simulink model "step_response_torque"  (R2024b)
settings: Solver=FixedStepAuto  StartTime=0.0  StopTime=10  FixedStep=Ts  RelTol=1e-3
values from neighbouring files (symbols this model uses):
  K_I = Ki_values(j)    [tune_PI_speed.m]
  K_p = Kp_values(i)    [tune_PI_speed.m]
  v0 = 10    [getItRunning.m]
libraries: slpidlib x1
settings Model: Creator=marti  LastModifiedBy=marti

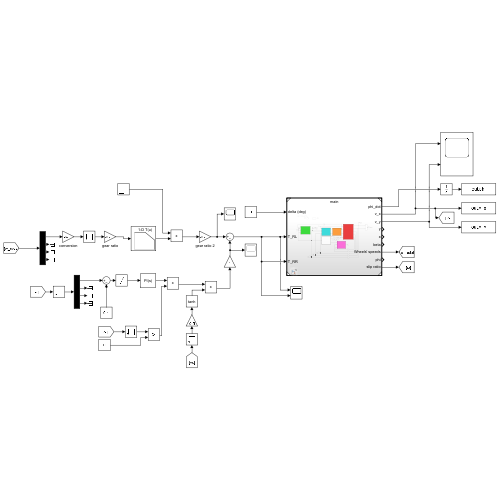
[thumbnail: Simulink's stored preview of the top-level diagram]
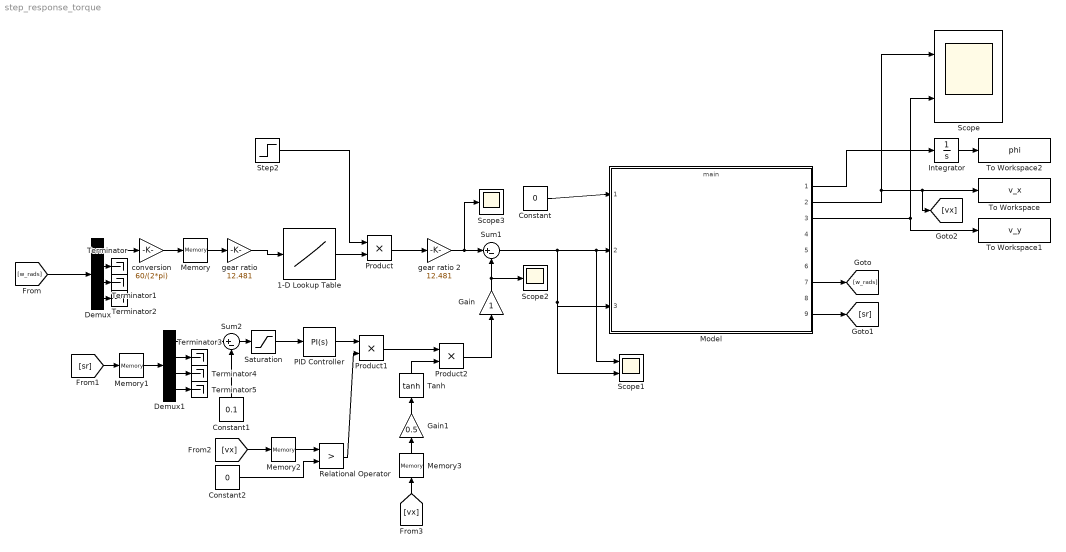
== system step_response_torque ==
  1-D Lookup Table : Lookup_n-D  NumberOfTableDimensions=1  BreakpointsForDimension1=[0;11400;19900;20000]  Table=[31.600000000000001;31.600000000000001;18;0]  InternalRulePriority=Speed  RndMeth=Simplest
  Constant : Constant  Value=0
  Constant1 : Constant  Value=0.1
  Constant2 : Constant  Value=0
  Demux : Demux
  Demux1 : Demux
  Gain : Gain
  Gain1 : Gain  Gain=0.5
  Integrator : Integrator
  Memory : Memory
  Memory1 : Memory
  Memory2 : Memory  InitialCondition=v0
  Memory3 : Memory  InitialCondition=v0
  Model : ModelReference  ModelNameDialog=main.slx  SimulationMode=Normal  ModelReferenceVersion=1.138
  PID Controller : slpidlib/PID Controller  Controller=PI  Form=Parallel  TimeDomain=Continuous-time  UseExternalTs=off  SampleTime=-1  IntegratorMethod=Forward Euler  FilterMethod=Forward Euler  ControllerParametersSource=internal  P=K_p  I=K_I  UseKiTs=off  D=0  UseExternalDerivativeSource=off  N=100  UseFilter=on  TunerSelectOption=Transfer Function Based (PID Tuner App)  InitialConditionSource=internal  InitialConditionForIntegrator=0  InitialConditionForFilter=0  DifferentiatorICPrevScaledInput=0  ExternalReset=none  TrackingMode=off  Kt=1  LimitOutput=off  SatLimitsSource=internal  UpperSaturationLimit=inf  LowerSaturationLimit=-inf  LinearizeAsGain=on  AntiWindupMode=none  Kb=1  LimitIntegrator=off  UpperIntegratorSaturationLimit=inf  LowerIntegratorSaturationLimit=-inf  POutMin=[]  POutMax=[]  IOutMin=[]  IOutMax=[]  DOutMin=[]  DOutMax=[]  NOutMin=[]  NOutMax=[]  SumOutMin=[]  SumOutMax=[]  SaturationOutMin=[]  SaturationOutMax=[]  PParamMin=[]  PParamMax=[]  IParamMin=[]  IParamMax=[]  DParamMin=[]  DParamMax=[]  NParamMin=[]  NParamMax=[]  KbParamMin=[]  KbParamMax=[]  KtParamMin=[]  KtParamMax=[]  KbOutMin=[]  KbOutMax=[]  KtOutMin=[]  KtOutMax=[]  IntegratorOutMin=[]  IntegratorOutMax=[]  FilterOutMin=[]  FilterOutMax=[]  SumI1OutMin=[]  SumI1OutMax=[]  SumI2OutMin=[]  SumI2OutMax=[]  SumI3OutMin=[]  SumI3OutMax=[]  SumI4OutMin=[]  SumI4OutMax=[]  SumDOutMin=[]  SumDOutMax=[]  DifferentiatorOutMin=[]  DifferentiatorOutMax=[]  FilterDiffOutCoefMin=[]  FilterDiffOutCoefMax=[]  ReciprocalOutMin=[]  ReciprocalOutMax=[]  SumDenOutMin=[]  SumDenOutMax=[]  SumNumOutMin=[]  SumNumOutMax=[]  DivideOutMin=[]  DivideOutMax=[]  UdiffTsProdOutMin=[]  UdiffTsProdOutMax=[]  NTsProdOutMin=[]  NTsProdOutMax=[]  UintegralTsProdOutMin=[]  UintegralTsProdOutMax=[]  UngainTsProdOutMin=[]  UngainTsProdOutMax=[]  ClampingZeroOutDataTypeStr=Inherit: Inherit via back propagation  ClampingZeroOutMin=[]  ClampingZeroOutMax=[]  FilterDenConstantOutDataTypeStr=Inherit: Inherit via back propagation  FilterDenConstantOutMin=[]  FilterDenConstantOutMax=[]  PCopyOutDataTypeStr=Inherit: Inherit via back propagation  PCopyOutMin=[]  PCopyOutMax=[]  NCopyOutDataTypeStr=Inherit: Inherit via back propagation  NCopyOutMin=[]  NCopyOutMax=[]  IntegratorContinuousStateAttributes=''  IntegratorStateMustResolveToSignalObject=off  IntegratorRTWStateStorageClass=Auto  FilterContinuousStateAttributes=''  FilterStateMustResolveToSignalObject=off  FilterRTWStateStorageClass=Auto  ParallelPVariant=InternalParameters  IdealPVariant=Disabled  IVariant=InternalParameters  DVariant=Disabled  IntegratorVariant=Continuous  SatVariant=Disabled  AWVariant=Passthrough  PCopyVariant=Disabled  TRVariant=Disabled  FdbkBlocksVariant=Forward  IdealPFdbkVariant=Disabled  SatFdbkVariant=Disabled  DerivativeFilterVariant=Disabled  NVariant=Disabled  NCopyVariant=Disabled_SignalSpec  FilterICVariant=Disabled  IntegratorICVariant=InternalICs  ExternalResetVariant=Disabled  TRSumVariant=Passthrough  SumFdbkVariant=Disabled  SumVariant=Sum_PI  TsampFilterVariant=InternalTs  TsampNgainVariant=Passthrough  TsampIntegralVariant=Disabled_SignalSpec  ExternalSaturationOutDataTypeStr=Inherit: Same as second input  DerivativeSourceVariant=Disabled  PreIntVariant=InternalPreInt
  Product : Product
  Product1 : Product
  Product2 : Product
  Relational Operator : RelationalOperator  Operator=>  OutDataTypeStr=boolean  RndMeth=Simplest  InputSameDT=off
  Saturation : Saturate  UpperLimit=inf  LowerLimit=0
  Scope : Scope  NumInputPorts=2
  Scope1 : Scope  NumInputPorts=2
  Scope2 : Scope
  Scope3 : Scope
  Step2 : Step  Time=2  SampleTime=0
  Sum1 : Sum  Inputs=|+-
  Sum2 : Sum  Inputs=|+-
  Tanh : Trigonometry  Operator=tanh
  Terminator{,1..5} (6 alike) : Terminator
  To Workspace : ToWorkspace  VariableName=v_x  SaveFormat=Structure With Time  SampleTime=-1
  To Workspace1 : ToWorkspace  VariableName=v_y  SaveFormat=Structure With Time  SampleTime=-1
  To Workspace2 : ToWorkspace  VariableName=phi  SaveFormat=Structure With Time  SampleTime=-1
  conversion : Gain  Gain=60/(2*pi)
  gear ratio : Gain  Gain=12.481
  gear ratio 2 : Gain  Gain=12.481
  wires:
  Constant/1 -> Model/1
  Model/3 -> To Workspace1/1, Scope/2
  Integrator/1 -> To Workspace2/1
  Model/1 -> Integrator/1
  Model/7 -> [w_rads]
  Demux/1 -> conversion/1
  Product/1 -> gear ratio 2/1
  Demux/4 -> Terminator2/1
  Demux/3 -> Terminator1/1
  conversion/1 -> Memory/1
  gear ratio/1 -> 1-D Lookup Table/1
  1-D Lookup Table/1 -> Product/2
  Demux/2 -> Terminator/1
  Memory/1 -> gear ratio/1
  [w_rads] -> Demux/1
  Model/9 -> [sr]
  [sr] -> Memory1/1
  Demux1/3 -> Terminator4/1
  Demux1/4 -> Terminator5/1
  gear ratio 2/1 -> Scope3/1, Sum1/1
  Demux1/2 -> Terminator3/1
  Sum2/1 -> Saturation/1
  Demux1/1 -> Sum2/1
  Constant1/1 -> Sum2/2
  Sum1/1 -> Model/3, Scope1/2, Scope1/1, Model/2
  Saturation/1 -> PID Controller/1
  Memory1/1 -> Demux1/1
  Gain/1 -> Scope2/1, Sum1/2
  Model/2 -> Scope/1, [vx], To Workspace/1
  [vx] -> Memory2/1
  Constant2/1 -> Relational Operator/2
  Memory2/1 -> Relational Operator/1
  Step2/1 -> Product/1
  PID Controller/1 -> Product1/1
  Relational Operator/1 -> Product1/2
  [vx] -> Memory3/1
  Memory3/1 -> Gain1/1
  Product1/1 -> Product2/1
  Tanh/1 -> Product2/2
  Product2/1 -> Gain/1
  Gain1/1 -> Tanh/1
